simulink model "G7221"  (Simulink 7.8)
settings: Solver=ode45  StartTime=0.0  StopTime=2  RelTol=1e-3
values from neighbouring files (symbols this model uses):
  g0 = h0    [G722_1.m]    (also in audio_test1.m = gsy(:,1); audio_test2.m = gsy(:,1))
  g1 = fliplr(h1)    [G722_1.m]    (also in audio_test1.m = gsy(:,2); audio_test2.m = gsy(:,2))
  h0 = zeros(1,L)    [G722_1.m]    (also in audio_test1.m = han(:,1); audio_test2.m = han(:,1); band4.m = fir1(nf, 2*ftp))
  h1 = firpm(128,f,m)    [CFIR_1.m]    (also in G722_1.m = (-1).^(0:L-1).*h0; audio_test1.m = han(:,2); audio_test2.m = han(:,2))
  Ts = 1/fs    (= 6.25e-05)    [G722_1.m]    (also in adaptiv_2.m = 0.001; adaptiv_3.m = 0.001; adaptiv_4.m = 0.001; adaptiv_5.m = 0.001)
libraries: dspsigops x5, dsparch4 x1
settings Model: Creator=svenhoffmann  LastModifiedBy=josef  ExtModeAutoUpdateStatusClock=off
settings DataIOCC: SignalLoggingName=sigsOut
settings OptimizationCC: InitFltsAndDblsToZero=on
settings DebuggingCC: SaveWithParameterizedLinksMsg=none  SignalResolutionControl=TryResolveAllWithWarning  SolverPrmCheckMsg=none  MultiTaskDSMMsg=warning  MultiTaskCondExecSysMsg=none  FcnCallInpInsideContextMsg=Use local settings  StrictBusMsg=None
settings HardwareCC: TargetUnknown=on
settings RTWCC: IncludeERTFirstTime=on
settings GRTTargetCC: TargetFcnLib=ansi_tfl_tmw.mat

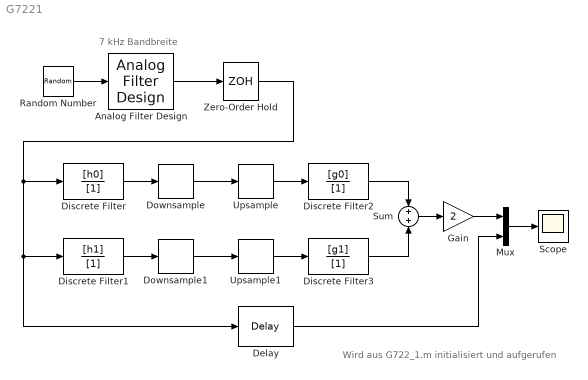
== system G7221 ==
  note: 7 kHz Bandbreite
  note: Wird aus G722_1.m initialisiert und aufgerufen
  Analog Filter Design : dsparch4/Analog Filter Design  method=Chebyshev I  filttype=Lowpass  N=8  Wlo=2*pi*7000  Whi=80  Rp=2  Rs=40
  Delay : dspsigops/Delay  InputProcessing=Inherited (this choice will be removed - see release notes)  dly_unit=Samples  delay=23  ic_detail=off  dif_ic_for_ch=off  dif_ic_for_dly=off  ic=0  reset_popup=None
  Discrete Filter : DiscreteFilter  Numerator=[h0]  Denominator=[1]  SampleTime=Ts
  Discrete Filter1 : DiscreteFilter  Numerator=[h1]  Denominator=[1]  SampleTime=Ts
  Discrete Filter2 : DiscreteFilter  Numerator=[g0]  Denominator=[1]  SampleTime=Ts
  Discrete Filter3 : DiscreteFilter  Numerator=[g1]  Denominator=[1]  SampleTime=Ts
  Downsample : dspsigops/Downsample  N=2  phase=0  InputProcessing=Inherited (this choice will be removed - see release notes)  RateOptions=Enforce single-rate processing  smode=Allow multirate  fmode=Maintain input frame size  ic=0
  Downsample1 : dspsigops/Downsample  N=2  phase=0  InputProcessing=Inherited (this choice will be removed - see release notes)  RateOptions=Enforce single-rate processing  smode=Allow multirate  fmode=Maintain input frame size  ic=0
  Gain : Gain  Gain=2  SaturateOnIntegerOverflow=on  OutDataTypeStr=Inherit: Same as input  ParamDataTypeStr=Inherit: Same as input
  Mux : Mux  Inputs=2
  Random Number : RandomNumber  SampleTime=0
  Scope : Scope
  Sum : Sum  SaturateOnIntegerOverflow=on
  Upsample : dspsigops/Upsample  N=2  phase=0  InputProcessing=Inherited (this choice will be removed - see release notes)  RateOptions=Allow multirate processing  ic=0  mode=Unused parameter value
  Upsample1 : dspsigops/Upsample  N=2  phase=0  InputProcessing=Inherited (this choice will be removed - see release notes)  RateOptions=Allow multirate processing  ic=0  mode=Unused parameter value
  Zero-Order Hold : ZeroOrderHold  SampleTime=Ts
  wires:
  Discrete Filter/1 -> Downsample/1
  Discrete Filter1/1 -> Downsample1/1
  Downsample/1 -> Upsample/1
  Downsample1/1 -> Upsample1/1
  Upsample1/1 -> Discrete Filter3/1
  Upsample/1 -> Discrete Filter2/1
  Discrete Filter3/1 -> Sum/2
  Discrete Filter2/1 -> Sum/1
  Sum/1 -> Gain/1
  Mux/1 -> Scope/1
  Delay/1 -> Mux/2
  Gain/1 -> Mux/1
  Random Number/1 -> Analog Filter Design/1
  Analog Filter Design/1 -> Zero-Order Hold/1
  Zero-Order Hold/1 -> Discrete Filter/1, Discrete Filter1/1, Delay/1
